simulink model "L0103"  (R2022b)
settings: Solver=VariableStepAuto  StartTime=0.0  StopTime=10.0  RelTol=1e-3
settings Model: Creator=Andrey  LastModifiedBy=Andrey

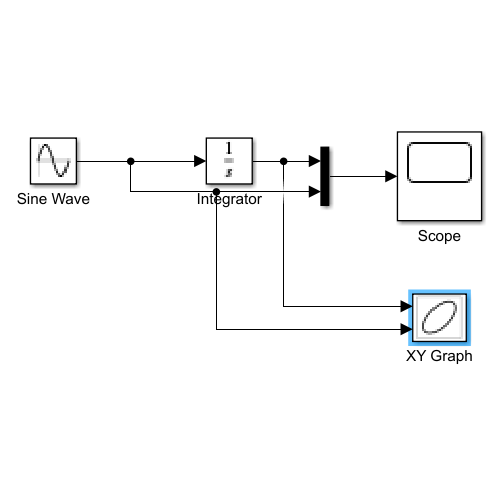
[thumbnail: Simulink's stored preview of the top-level diagram]
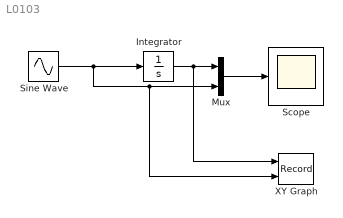
== system L0103 ==
  Integrator : Integrator
  Mux : Mux  Inputs=2
  Scope : Scope
  Sine Wave : Sin  SampleTime=0
  XY Graph : Record  FileSettingsInternal="{\"entries\":[{\"content\":{\"excelSettings\":{\"content\":{},\"type\":\"Streamout.ExcelSettings\"}},\"type\":\"Streamout.FileSettingStorage\",\"uuid\":\"c5ddcaae-fee7-4fa9-9aa8-a3297d4614a0\"}],\"packageUris\":[\"http://schema.mathworks.com/mf0/streamout_blocks/R2020a\"],\"version\":\"1.0\"}"  Layout=[1 1]  SignalsInternal="{\"entries\":[{\"content\":{\"signals\":[{\"content\":{\"blockPath\":[\"L0103/XY Graph\"],\"channel\":[],\"dimensions\":[1],\"domain\":\"L0103/XY Graph\",\"lineColor\":\"#a2142f\",\"plots\":[1],\"port\":1,\"sid\":[\"\"],\"signalID\":78,\"signalName\":\"Integrator\"},\"type\":\"RecordBlkView.Signal\",\"uuid\":\"3466af9a-dc45-4879-8e2d-b97faf7ba168\"},{\"content\":{\"blockPath\":[\"L0103/XY Graph\"],\"channel\":[],\"dimensions\":[1],\"domain\":\"L0103/XY Graph\",\"lineColor\":\"#139fff\",\"plots\":[1],\"port\":2,\"sid\":[\"\"],\"signalID\":82,\"signalName\":\"Sine Wave\"},\"type\":\"RecordBlkView.Signal\",\"uuid\":\"898c229a-33c6-4a6d-bbd3-6a86c8059bc6\"}]},\"type\":\"RecordBlkView.InputSignals\",\"uuid\":\"6430f203-0ef9-4975-999b-435d22915f8d\"}],\"packageUris\":[\"http://schema.mathworks.com/mf0/streamout_blocks/R2020a\"],\"version\":\"1.0\"}"  VisualizationBindings="{\"xyplotplugin\":{\"info\":[{\"series\":[{\"bindingParametersList\":[{\"parameter\":\"X-Axis\",\"signalID\":78,\"signalName\":\"Integrator\"},{\"parameter\":\"Y-Axis\",\"signalID\":82,\"signalName\":\"Sine Wave\"}],\"seriesID\":41294}],\"subplotID\":1}]}}"  CompatibilityTag=XY
  wires:
  Sine Wave/1 -> XY Graph/2, Mux/2, Integrator/1
  Mux/1 -> Scope/1
  Integrator/1 -> XY Graph/1, Mux/1
